simulink model "pair_sched_lqr"  (R2025b)
settings: Solver=ode45  StartTime=0.0  StopTime=10  MaxStep=0.005  RelTol=1e-3
InitFcn:
  | addpath(fileparts(get_param(bdroot, 'FileName')))
settings Model: Creator=derekg  LastModifiedBy=derekg

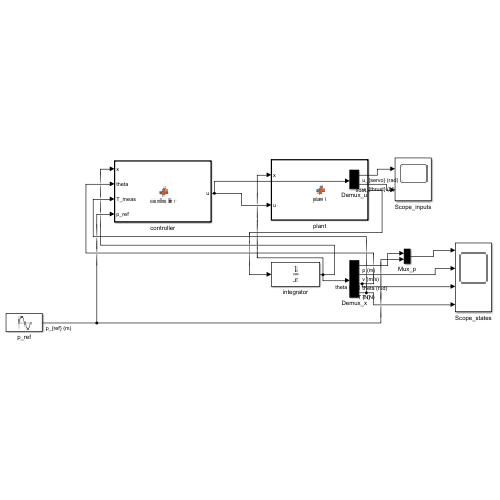
[thumbnail: Simulink's stored preview of the top-level diagram]
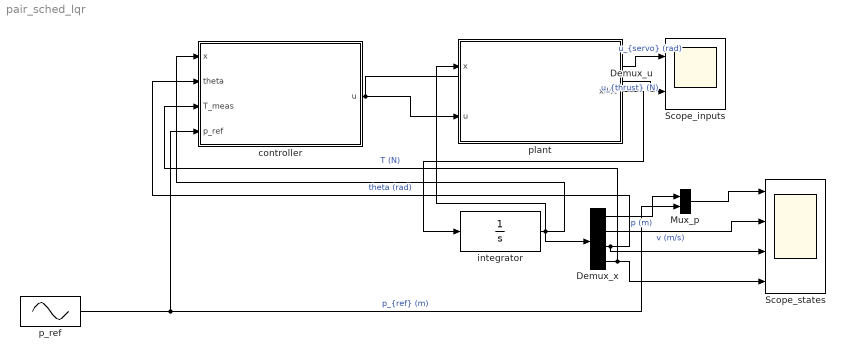
== system pair_sched_lqr ==
  Demux_u : Demux  Outputs=2
  Demux_x : Demux
  Mux_p : Mux  Inputs=2
  Scope_inputs : Scope  NumInputPorts=2
  Scope_states : Scope  NumInputPorts=4
      settings: ActiveDisplayYMinimum=-0.57642868660175983  ActiveDisplayYMaximum=0.43211387221916553
  controller : MATLAB Function  TreatAsAtomicUnit=on
  integrator : Integrator  InitialCondition=[0; 0; 0; 2.574]
  p_ref : Sin  Amplitude=.15  Frequency=2  SampleTime=0
  plant : MATLAB Function  TreatAsAtomicUnit=on
  wires:
  integrator/1 -> controller/1(x), plant/1(x), Demux_x/1
  Demux_x/3 -> controller/2(theta), Scope_states/3  "theta (rad)"
  Demux_x/4 -> controller/3(T_meas), Scope_states/4  "T (N)"
  p_ref/1 -> controller/4(p_ref), Mux_p/2  "p_{ref} (m)"
  controller/1(u) -> plant/2(u), Demux_u/1
  plant/1(xdot) -> integrator/1
  Demux_x/1 -> Mux_p/1  "p (m)"
  Mux_p/1 -> Scope_states/1
  Demux_x/2 -> Scope_states/2  "v (m/s)"
  Demux_u/1 -> Scope_inputs/1  "u_{servo} (rad)"
  Demux_u/2 -> Scope_inputs/2  "u_{thrust} (N)"

== matlab function pair_sched_lqr/plant ==
  data: x input; u input; xdot output
function xdot = plant(x, u)
% Nonlinear EOM: x = [p; v; theta; T],  u = [theta_cmd_rad; T_cmd_N]
m          = 0.4536;
tau_servo  = 0.0244;
tau_thrust = 0.0781;
mu_c       = 0.8158;
v_sign = tanh(x(2) / 0.05);   % smooth sign: avoids chattering at v≈0 (ε = 5 mm/s)
xdot = [x(2);
        (x(4)*sin(x(3)) - mu_c*v_sign) / m;
        (u(1) - x(3)) / tau_servo;
        (u(2) - x(4)) / tau_thrust];
end

== matlab function pair_sched_lqr/controller ==
  data: x input; u output; theta input; T_meas input; p_ref input
function u = controller(x, theta, T_meas, p_ref)
% Pair-scheduled LQR. K(theta, T) interpolated from 2D gain table using live states.
% Scheduling variables are x(3) (servo angle) and x(4) (thrust).
% Control law: u = u_star - K * (x - x_star),  x_star(1) = p_ref
persistent theta_s T_s K_s
if isempty(theta_s)
    tmp     = coder.load('gain_schedule_tier3.mat');
    theta_s = tmp.theta_sched;
    T_s     = tmp.T_sched;
    K_s     = tmp.K_sched;
end
K = zeros(2, 4);
for i = 1:2
    for j = 1:4
        K(i,j) = interp2(T_s, theta_s, squeeze(K_s(i,j,:,:)), T_meas, theta, 'linear');
    end
end
T_nom  = 2.574;
x_star = [p_ref; 0; 0; T_nom];
u_star = [0; T_nom];
u = u_star - K * (x - x_star);
u(1) = max(min(u(1), pi/3), -pi/3);  % servo ±60°
u(2) = max(min(u(2), 4.17), 0);      % thrust 0–4.17 N (static sweep at 1950 µs)
end
